simulink model "App_code"  (R2022b)
settings: Solver=FixedStepDiscrete  StartTime=0.0  StopTime=10.0  FixedStep=0.01  RelTol=1e-3
undefined symbols (not defined in the file or in its folder): App_modes
settings Model: ExtModeTrigDuration=2  Creator=Dell  LastModifiedBy=Dell
settings OptimizationCC: DefaultParameterBehavior=Inlined  UseDivisionForNetSlopeComputation=on  GainParamInheritBuiltInType=on  UseFloatMulNetSlope=on  InlineInvariantSignals=on  PassReuseOutputArgsAs=Individual arguments  ZeroExternalMemoryAtStartup=off  ZeroInternalMemoryAtStartup=off  NoFixptDivByZeroProtection=on  EfficientFloat2IntCast=on  LifeSpan=1  MaxStackSize=64  OptimizeBlockOrder=speed  DifferentSizesBufferReuse=on  EfficientTunableParamExpr=on
settings DebuggingCC: ParameterTunabilityLossMsg=error
settings HardwareCC: ProdBitPerInt=16  ProdBitPerPointer=16  ProdBitPerSizeT=16  ProdBitPerPtrDiffT=16  ProdLargestAtomicFloat=None  ProdWordSize=8  ProdLongLongMode=on  ProdHWDeviceType=Atmel->AVR
settings SFSimCC: MATLABDynamicMemAlloc=off
settings RTWCC: Description=Embedded Coder  SystemTargetFile=ert.tlc  HardwareBoard=Arduino Uno  TLCOptions=-aInlineSetEventsForThisBaseRateFcn=TLC_FALSE -aSuppressMultiTaskScheduler=TLC_FALSE -aRateBasedStepFcn=1  TemplateMakefile=ert_default_tmf  Toolchain=Arduino AVR  BuildConfiguration=Faster Runs
settings CodeAppCC: ForceParamTrailComments=on  IgnoreCustomStorageClasses=off  OperatorAnnotations=on  SimulinkDataObjDesc=on  SFDataObjDesc=on  CustomSymbolStrGlobalVar=rt$N$M  CustomSymbolStrType=$N$M  CustomSymbolStrFcn=$N$M$F  CustomSymbolStrMacro=$N$M  InsertBlockDesc=on
settings ERTTargetCC: IncludeMdlTerminateFcn=off  CombineSignalStateStructs=on  SuppressErrorStatus=on  SupportAbsoluteTime=off  SupportComplex=off  ExtModeTransport=3  ExtModeStaticAlloc=on  ExtModeAutomaticAllocSize=off  ExtModeStaticAllocSize=250  ExtModeMexFile=ext_xcp  ExtModeIntrfLevel=Level2 - Open  InlinedParameterPlacement=NonHierarchical  ERTFilePackagingFormat=CompactWithDataFile

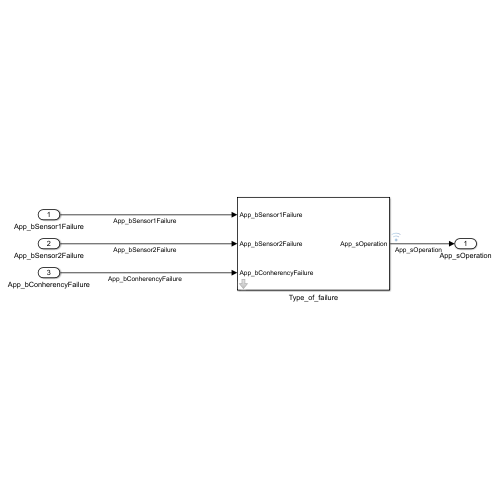
[thumbnail: Simulink's stored preview of the top-level diagram]
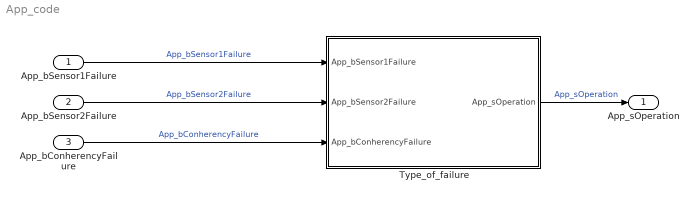
== system App_code ==
  App_bSensor1Failure : Inport
  App_bSensor2Failure : Inport  Port=2
  App_bConherencyFailure : Inport  Port=3
  Type_of_failure : Subsystem  InitFcn=init
  App_sOperation : Outport
  wires:
  Type_of_failure/1(App_sOperation) -> App_sOperation/1  "App_sOperation"
  App_bSensor1Failure/1 -> Type_of_failure/1(App_bSensor1Failure)  "App_bSensor1Failure"
  App_bSensor2Failure/1 -> Type_of_failure/2(App_bSensor2Failure)  "App_bSensor2Failure"
  App_bConherencyFailure/1 -> Type_of_failure/3(App_bConherencyFailure)  "App_bConherencyFailure"

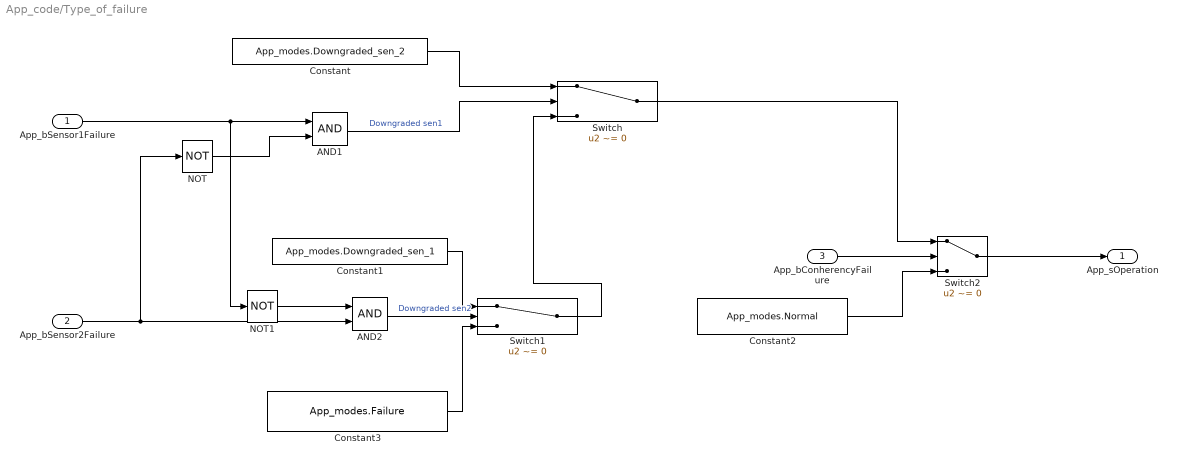
== system App_code/Type_of_failure ==
  App_bSensor1Failure : Inport
  App_bSensor2Failure : Inport  Port=2
  App_bConherencyFailure : Inport  Port=3
  AND1 : Logic  AllPortsSameDT=off  OutDataTypeStr=boolean
  AND2 : Logic  AllPortsSameDT=off  OutDataTypeStr=boolean
  Constant : Constant  Value=App_modes.Downgraded_sen_2  OutDataTypeStr=Enum: App_modes
  Constant1 : Constant  Value=App_modes.Downgraded_sen_1  OutDataTypeStr=Enum: App_modes
  Constant2 : Constant  Value=App_modes.Normal  OutDataTypeStr=Enum: App_modes
  Constant3 : Constant  Value=App_modes.Failure  OutDataTypeStr=Enum: App_modes
  NOT : Logic  Operator=NOT  IconShape=distinctive  AllPortsSameDT=off  OutDataTypeStr=boolean
  NOT1 : Logic  Operator=NOT  IconShape=distinctive  AllPortsSameDT=off  OutDataTypeStr=boolean
  Switch : Switch  Criteria=u2 ~= 0  SaturateOnIntegerOverflow=off  InputSameDT=off
  Switch1 : Switch  Criteria=u2 ~= 0  SaturateOnIntegerOverflow=off  InputSameDT=off
  Switch2 : Switch  Criteria=u2 ~= 0  SaturateOnIntegerOverflow=off  InputSameDT=off
  App_sOperation : Outport  OutDataTypeStr=Enum: App_modes  LockScale=on
  wires:
  NOT/1 -> AND1/2
  NOT1/1 -> AND2/1
  App_bSensor1Failure/1 -> NOT1/1, AND1/1
  App_bSensor2Failure/1 -> NOT/1, AND2/2
  AND1/1 -> Switch/2  "Downgraded sen1"
  AND2/1 -> Switch1/2  "Downgraded sen2"
  Switch/1 -> Switch2/1
  Switch2/1 -> App_sOperation/1
  App_bConherencyFailure/1 -> Switch2/2
  Switch1/1 -> Switch/3
  Constant/1 -> Switch/1
  Constant2/1 -> Switch2/3
  Constant1/1 -> Switch1/1
  Constant3/1 -> Switch1/3
